simulink model "GDFLIB_FilterMA_BAM_F32"  (Simulink 7.3)
settings: Solver=ode45  StartTime=0.0  StopTime=10.0  RelTol=1e-3
undefined symbols (not defined in the file): u16NSamples
settings Model: Creator=RE004C  LastModifiedBy=RE004C
settings HardwareCC: ProdIntDivRoundTo=Zero  ProdEndianess=BigEndian  ProdHWDeviceType=Freescale->32-bit PowerPC

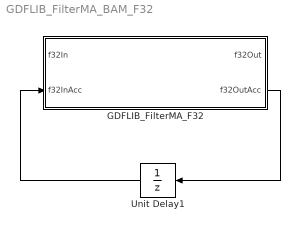
== system GDFLIB_FilterMA_BAM_F32 ==
  GDFLIB_FilterMA_F32 : Subsystem  mask(GDFLIB_FilterMA_F32){u16NSamples=u16NSamples}
      mask help: Bit accurate model of recursive form moving average filter. All parameters as well as input and output are 32bit integers.
      mask init:
      | pos = get_param(gcb, 'Position');width = pos(3) - pos(1); height = pos(4) - pos(2);tX=width/2;tY=height*0.9;
      mask Display:
      | color('black');
      | port_label('input',1,'f32In');
      | port_label('input',2,'f32InAcc');
      | port_label('output',1,'f32Out');
      | port_label('output',2,'f32OutAcc');
      | color('black');
      | disp('GDFLIB_FilterMA_F32');
      | color('blue');
      | text(tX,tY, 'BAM', 'horizontalAlignment', 'center');
  Unit Delay1 : UnitDelay  SampleTime=-1
  wires:
  GDFLIB_FilterMA_F32/2(f32OutAcc) -> Unit Delay1/1
  Unit Delay1/1 -> GDFLIB_FilterMA_F32/2(f32InAcc)

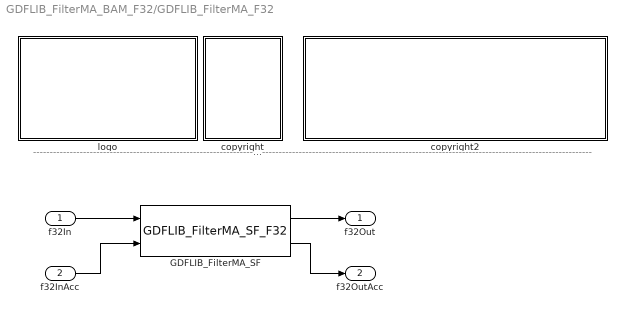
== system GDFLIB_FilterMA_BAM_F32/GDFLIB_FilterMA_F32 ==
  note: ---------------------------------------------------------------------------------------------------------------------------------------------------------------------------------------------------
  f32In : Inport  OutDataType=fixdt(1, 16)  OutScaling=2^0
  f32InAcc : Inport  Port=2  OutDataType=fixdt(1, 16)  OutScaling=2^0
  GDFLIB_FilterMA_SF : S-Function  FunctionName=GDFLIB_FilterMA_SF_F32  Parameters=u16NSamples  EnableBusSupport=off
  copyright : Subsystem
      mask Display: text(10,90,'FILE:');text(10,75,'DESRIPTION:')text(10,60,'COPYRIGHT:')text(10,45,'VERSION:')text(10,30,'DATE:')
  copyright2 : Subsystem
      mask Display: text(10,90,'GDFLIB_FilterMA_BAM_F32.mdl');text(10,75,'Recursive form moving average filter.');text(10,60,'Freescale')text(10,45,'0.1');text(10,30,'16-Jan-2012');
  logo : Subsystem
      mask Display: image(imread('logo.jpg'))
  f32Out : Outport  OutDataType=fixdt(1, 16)  OutScaling=2^0
  f32OutAcc : Outport  Port=2  OutDataType=fixdt(1, 16)  OutScaling=2^0
  wires:
  f32In/1 -> GDFLIB_FilterMA_SF/1
  GDFLIB_FilterMA_SF/1 -> f32Out/1
  f32InAcc/1 -> GDFLIB_FilterMA_SF/2
  GDFLIB_FilterMA_SF/2 -> f32OutAcc/1

== system GDFLIB_FilterMA_BAM_F32/GDFLIB_FilterMA_F32/copyright ==

== system GDFLIB_FilterMA_BAM_F32/GDFLIB_FilterMA_F32/copyright2 ==

== system GDFLIB_FilterMA_BAM_F32/GDFLIB_FilterMA_F32/logo ==
